simulink model "Controller"  (R2024a)
settings: Solver=VariableStepAuto  StartTime=0.0  StopTime=10  RelTol=1e-3
model workspace (MAT data in the model file):
  Ts = 0.1
  ki = 1
  kp = 0.2
settings Model: Creator=awabm  LastModifiedBy=awabm

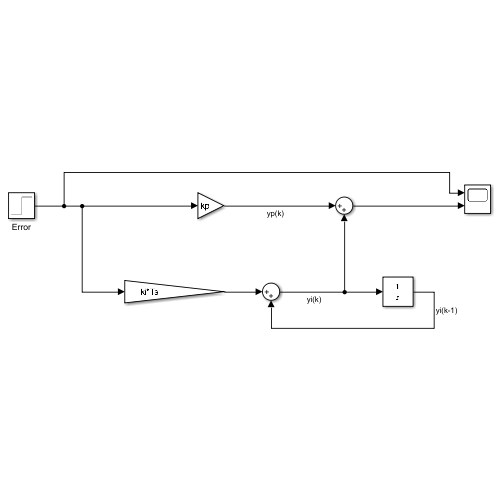
[thumbnail: Simulink's stored preview of the top-level diagram]
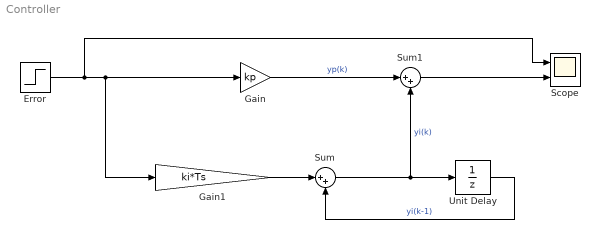
== system Controller ==
  Error : Step  SampleTime=0.1
  Gain : Gain  Gain=kp
  Gain1 : Gain  Gain=ki*Ts
  Scope : Scope  NumInputPorts=2
  Sum : Sum  Inputs=|++
  Sum1 : Sum  Inputs=|++
  Unit Delay : UnitDelay  SampleTime=Ts  HasFrameUpgradeWarning=on
  wires:
  Error/1 -> Scope/1, Gain1/1, Gain/1
  Unit Delay/1 -> Sum/2  "yi(k-1)"
  Gain/1 -> Sum1/1  "yp(k)"
  Sum/1 -> Sum1/2, Unit Delay/1  "yi(k)"
  Sum1/1 -> Scope/2
  Gain1/1 -> Sum/1
